simulink model "TST_BusSelectorProblem"  (Simulink 10.0)
settings: Solver=FixedStepDiscrete  StartTime=0.0  StopTime=10.0  FixedStep=0.02  RelTol=1e-3  EnableMultiTasking=on
settings Model: Creator=kharthforeign  LastModifiedBy=unknown
settings DataIOCC: LimitDataPoints=on  SignalLoggingSaveFormat=ModelDataLogs  SaveOutput=off  SignalLogging=off  SaveTime=off
settings OptimizationCC: BlockReduction=off  ConditionallyExecuteInputs=off  OptimizeBlockIOStorage=off  BufferReuse=off  GlobalBufferReuse=off  ExpressionFolding=off  ExpressionDepthLimit=2147483647  LocalBlockOutputs=off  InitFltsAndDblsToZero=on  OptimizeDataStoreBuffers=off  BusAssignmentInplaceUpdate=off
settings DebuggingCC: SolverPrmCheckMsg=warning  FcnCallInpInsideContextMsg=warning  StateNameClashWarn=warning
settings GRTTargetCC: GeneratePreprocessorConditionals=Disable all
settings ConfigComp: CovExternalEMLEnable=off

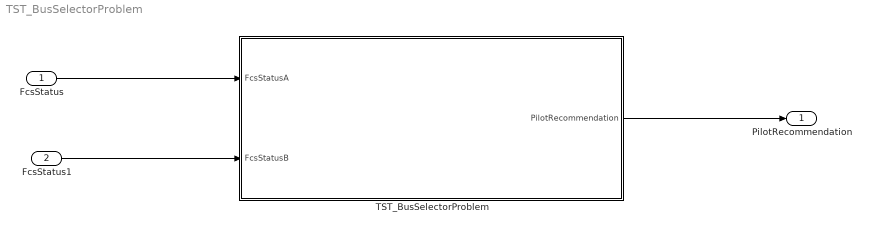
== system TST_BusSelectorProblem ==
  FcsStatus : Inport  OutDataTypeStr=Bus: FCS_FlightControlSystem_Status
  FcsStatus1 : Inport  Port=2  OutDataTypeStr=Bus: FCS_FlightControlSystem_Status
  TST_BusSelectorProblem : Subsystem  TreatAsAtomicUnit=on
  PilotRecommendation : Outport  OutDataTypeStr=uint32  PortDimensions=1
  wires:
  FcsStatus/1 -> TST_BusSelectorProblem/1(FcsStatusA)
  TST_BusSelectorProblem/1(PilotRecommendation) -> PilotRecommendation/1
  FcsStatus1/1 -> TST_BusSelectorProblem/2(FcsStatusB)

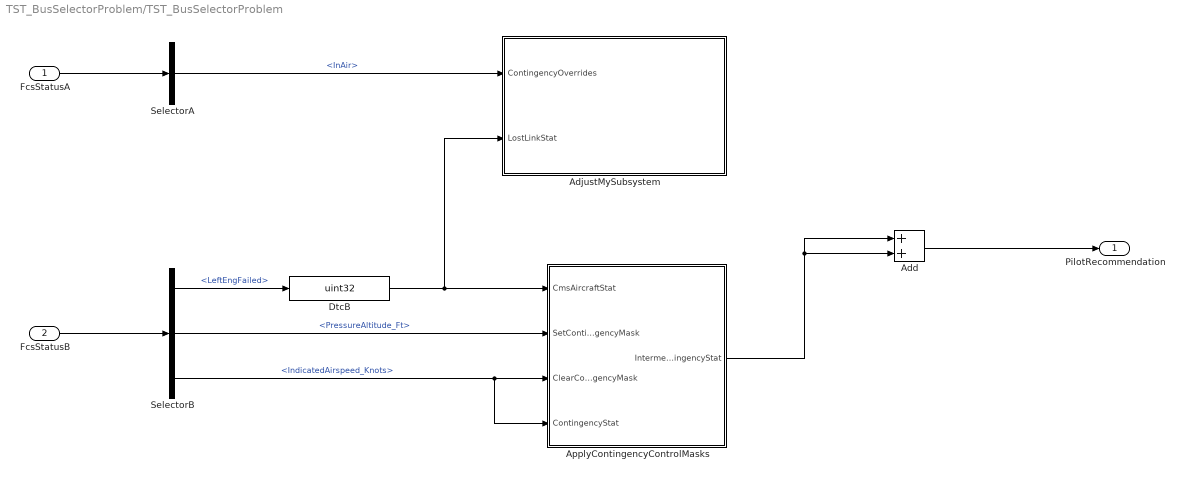
== system TST_BusSelectorProblem/TST_BusSelectorProblem ==
  FcsStatusA : Inport  OutDataTypeStr=Bus: FCS_FlightControlSystem_Status
  FcsStatusB : Inport  Port=2  OutDataTypeStr=Bus: FCS_FlightControlSystem_Status
  Add : Sum
  AdjustMySubsystem : Subsystem  TreatAsAtomicUnit=on
  ApplyContingencyControlMasks : Subsystem  TreatAsAtomicUnit=on
  DtcB : DataTypeConversion  OutDataTypeStr=uint32
  SelectorA : BusSelector  OutputSignals=InAir
  SelectorB : BusSelector  OutputSignals=LeftEngFailed,PressureAltitude_Ft,IndicatedAirspeed_Knots
  PilotRecommendation : Outport  OutDataTypeStr=uint32  PortDimensions=1
  wires:
  FcsStatusA/1 -> SelectorA/1
  FcsStatusB/1 -> SelectorB/1
  SelectorA/1 -> AdjustMySubsystem/1(ContingencyOverrides)  "<InAir>"
  SelectorB/1 -> DtcB/1  "<LeftEngFailed>"
  DtcB/1 -> AdjustMySubsystem/2(LostLinkStat), ApplyContingencyControlMasks/1(CmsAircraftStat)
  SelectorB/2 -> ApplyContingencyControlMasks/2(SetContingencyMask)  "<PressureAltitude_Ft>"
  SelectorB/3 -> ApplyContingencyControlMasks/3(ClearContingencyMask), ApplyContingencyControlMasks/4(ContingencyStat)  "<IndicatedAirspeed_Knots>"
  Add/1 -> PilotRecommendation/1
  ApplyContingencyControlMasks/1(IntermediateContingencyStat) -> Add/2, Add/1

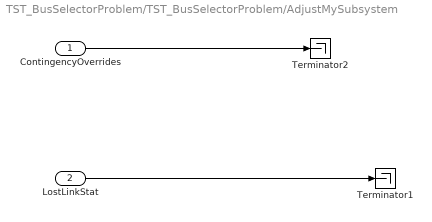
== system TST_BusSelectorProblem/TST_BusSelectorProblem/AdjustMySubsystem ==
  ContingencyOverrides : Inport
  LostLinkStat : Inport  Port=2
  Terminator1 : Terminator
  Terminator2 : Terminator
  wires:
  ContingencyOverrides/1 -> Terminator2/1
  LostLinkStat/1 -> Terminator1/1

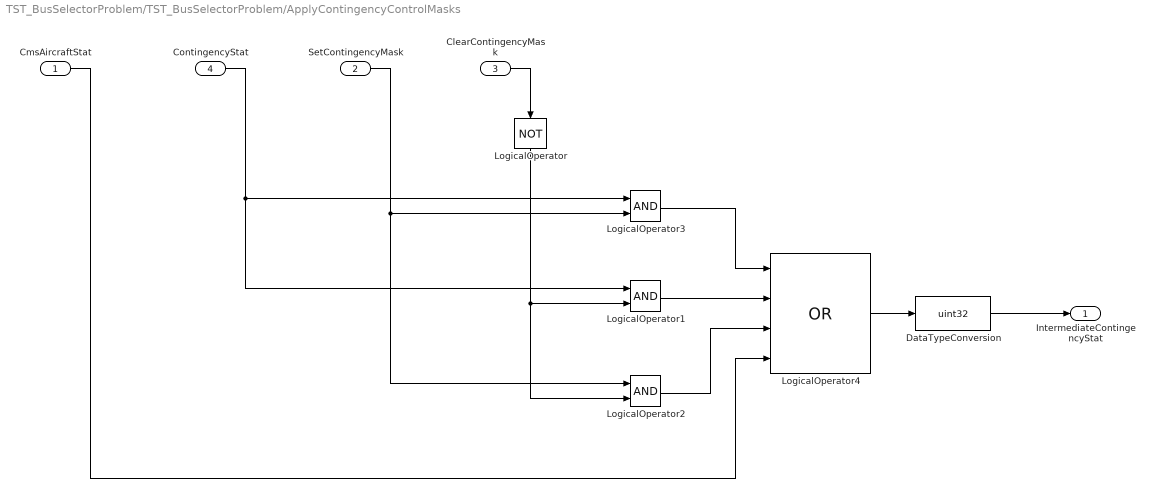
== system TST_BusSelectorProblem/TST_BusSelectorProblem/ApplyContingencyControlMasks ==
  CmsAircraftStat : Inport
  SetContingencyMask : Inport  Port=2
  ClearContingencyMask : Inport  Port=3
  ContingencyStat : Inport  Port=4
  DataTypeConversion : DataTypeConversion  OutDataTypeStr=uint32
  LogicalOperator : Logic  Operator=NOT  AllPortsSameDT=off  OutDataTypeStr=boolean
  LogicalOperator1 : Logic  AllPortsSameDT=off  OutDataTypeStr=boolean
  LogicalOperator2 : Logic  AllPortsSameDT=off  OutDataTypeStr=boolean
  LogicalOperator3 : Logic  AllPortsSameDT=off  OutDataTypeStr=boolean
  LogicalOperator4 : Logic  Operator=OR  Inputs=4  AllPortsSameDT=off  OutDataTypeStr=boolean
  IntermediateContingencyStat : Outport
  wires:
  LogicalOperator3/1 -> LogicalOperator4/1
  LogicalOperator1/1 -> LogicalOperator4/2
  LogicalOperator2/1 -> LogicalOperator4/3
  ClearContingencyMask/1 -> LogicalOperator/1
  SetContingencyMask/1 -> LogicalOperator2/1, LogicalOperator3/2
  LogicalOperator/1 -> LogicalOperator2/2, LogicalOperator1/2
  ContingencyStat/1 -> LogicalOperator1/1, LogicalOperator3/1
  CmsAircraftStat/1 -> LogicalOperator4/4
  LogicalOperator4/1 -> DataTypeConversion/1
  DataTypeConversion/1 -> IntermediateContingencyStat/1
